simulink model "MLP_Control_Of_Induction_Motor"  (R2025b)
settings: Solver=FixedStepAuto  StartTime=0.0  StopTime=7.5  FixedStep=Ts  MaxStep=1e-3  RelTol=1e-3  EnableMultiTasking=on
PreLoadFcn:
  | IMDriveSensorData
values from neighbouring files (symbols this model uses):
  fn = 50    [Model_and_motor_parameters_for_FOC.m]
  Ibase = Pn/(1.5*Vbase)    [Model_and_motor_parameters_for_FOC.m]
  Lm = 2.717    [Model_and_motor_parameters_for_FOC.m]
  p = 2    [Model_and_motor_parameters_for_FOC.m]
  Tbase = Pn/(wbase/p)    (= 1044.05642668)    [Model_and_motor_parameters_for_FOC.m]
  Ts = 5e-6    (= 5e-06)    [Model_and_motor_parameters_for_FOC.m]
  Tsc = 1/(fsw*10)    (= 5e-05)    [Model_and_motor_parameters_for_FOC.m]
  Vbase = Vn/sqrt(3)*sqrt(2)    [Model_and_motor_parameters_for_FOC.m]
  Xls = Lls*Zbase    [Model_and_motor_parameters_for_FOC.m]
undefined symbols (not defined in the file or in its folder): ee
libraries: nesl_utility x11, ee_lib x8, fl_lib x5, eePwmGeneratorTwoLevel x1, eeTransforms x1, eeAsmFluxObserver x1, SignalEditorBlockLib x1
CloseFcn:
  | clear simlog_IMDriveSensor
  | clear logsout_IMDriveSensor
Description:
  | Three-Phase Asynchronous Drive with Sensor Control
settings Model: SimulationMode=accelerator  Creator=The MathWorks, Inc.  LastModifiedBy=Harish
settings SolverCC: AlgebraicLoopSolver=TrustRegion  AutoInsertRateTranBlk=on
settings DataIOCC: MaxDataPoints=510000  SaveOperatingPoint=on  SaveFormat=StructureWithTime  SaveOutput=off  SaveTime=off  ReturnWorkspaceOutputs=off
settings OptimizationCC: ReuseModelBlockBuffer=off  ExpressionDepthLimit=2147483647.0  LifeSpan=inf
settings DebuggingCC: AlgebraicLoopMsg=error  UnderspecifiedInitializationDetection=Classic  MergeDetectMultiDrivingBlocksExec=none  SolverPrmCheckMsg=warning  MultiTaskRateTransMsg=warning  UnconnectedInputMsg=warning  UnconnectedOutputMsg=warning  UnconnectedLineMsg=warning  StateNameClashWarn=warning  SFUnexpectedBacktrackingDiag=warning  SFNoUnconditionalDefaultTransitionDiag=warning  SFExecutionAtInitializationDiag=none  ArithmeticOperatorsInVariantConditions=warning
settings HardwareCC: ProdBitPerPointer=32.0  ProdBitPerSizeT=32.0  ProdBitPerPtrDiffT=32.0  ProdLargestAtomicFloat=None  ProdIntDivRoundTo=Undefined  ProdEndianess=Unspecified  ProdWordSize=32.0  ProdHWDeviceType=32-bit Generic
settings ModelReferenceCC: EnableRefExpFcnMdlSchedulingChecks=on  PropagateSignalLabelsOutOfModel=off
settings SFSimCC: SimUseLocalCustomCode=off  CustomCodeUndefinedFunction=UseInterfaceOnly
settings RTWCC: RTWUseLocalCustomCode=off  GPUComputeCapability=3.5  DLArmComputeVersion=19.05
settings CodeAppCC: StateflowObjectComments=on
settings GRTTargetCC: TargetLangStandard=C89/C90 (ANSI)
settings ConfigComp: CovMetricSettings=dw  CovSaveCumulativeToWorkspaceVar=on  CovSaveSingleToWorkspaceVar=on  CovExternalEMLEnable=off  CovSFcnEnable=off
settings SimscapeCC: SimscapeLogType=all  SimscapeLogSimulationStatistics=on  SimscapeLogName=simlog_IMDriveSensor  SimscapeLogDecimation=5.0  SimscapeLogLimitData=off  SimscapeLogDataHistory=510000.0

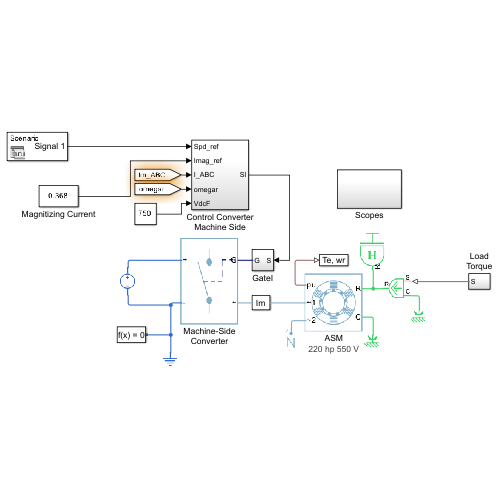
[thumbnail: Simulink's stored preview of the top-level diagram]
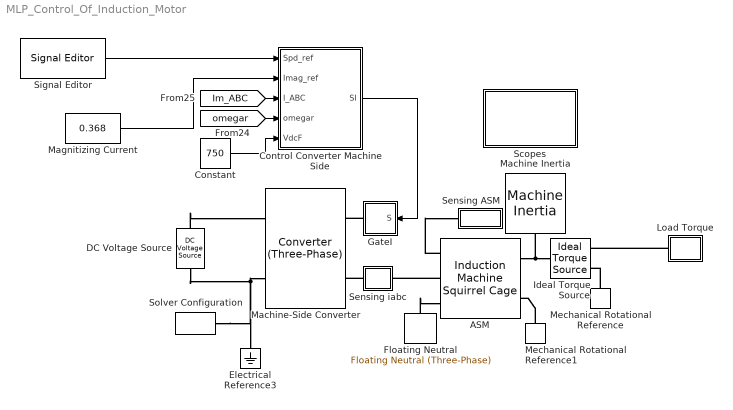
== system MLP_Control_Of_Induction_Motor ==
  ASM : ee_lib/Electromechanical/Asynchronous/Induction Machine Squirrel Cage  port_option=ee.enum.threePhasePort.composite  SRated=Pn V*A  VRated=Vn V  FRated=fn Hz  nPolePairs=p  param_unit=ee.enum.unit.si  squirrel_cage=ee.enum.squirrelcage.Single  zero_sequence=ee.enum.park.zerosequence.include  initialization_option=ee.enum.asm.initialization.fluxvariables  Rs=Rss Ohm  Xls=Xls Ohm  pu_Rs=0.0258  pu_Lls=0.0413  Rrd=Rrr Ohm  Xlrd=Xlr Ohm  pu_Rrd=0.0145  pu_Llrd=0.0424  Rrd1=0.28 Ohm  Xlrd1=0.82 Ohm  Rrd2=0.28 Ohm  Xlrd2=0.82 Ohm  pu_Rrd1=0.0290  pu_Llrd1=0.0848  pu_Rrd2=0.0290  pu_Llrd2=0.0848  Xm=Xm Ohm  pu_Lm=1.7562  X0=Xls Ohm  pu_L0=0.0413  saturation_option=0  saturation_i=[0, 4, 9, 18, 25, 34, 50, 68, 95, 120] A  saturation_v=[0, 88, 154, 198, 220, 242, 264, 286, 308, 330] V  pu_saturation_i=[0, .176, .396, .792, 1.1, 1.496, 2.2, 2.992, 4.18, 5.28]  pu_saturation_v=[0, .4, .7, .9, 1, 1.1, 1.2, 1.3, 1.4, 1.4864]  connection_option=int32(ee.enum.Connection.delta)  angular_position_specify=off  angular_position_priority=None  angular_position=0 deg  angular_position_nominal_specify=off  angular_position_nominal_value=1  angular_position_nominal_unit=deg  pu_psids_specify=off  pu_psids_priority=None  pu_psids=0  pu_psids_nominal_specify=off  pu_psids_nominal_value=1  pu_psids_nominal_unit=1  pu_psiqs_specify=off  pu_psiqs_priority=None  pu_psiqs=0  pu_psiqs_nominal_specify=off  pu_psiqs_nominal_value=1  pu_psiqs_nominal_unit=1  pu_psi0s_specify=off  pu_psi0s_priority=None  pu_psi0s=0  pu_psi0s_nominal_specify=off  pu_psi0s_nominal_value=1  pu_psi0s_nominal_unit=1  pu_psidr_specify=off  pu_psidr_priority=None  pu_psidr=0  pu_psidr_nominal_specify=off  pu_psidr_nominal_value=1  pu_psidr_nominal_unit=1  pu_psiqr_specify=off  pu_psiqr_priority=None  pu_psiqr=0  pu_psiqr_nominal_specify=off  pu_psiqr_nominal_value=1  pu_psiqr_nominal_unit=1  pu_psidr1_specify=off  pu_psidr1_priority=None  pu_psidr1=0  pu_psidr1_nominal_specify=off  pu_psidr1_nominal_value=1  pu_psidr1_nominal_unit=1  pu_psiqr1_specify=off  pu_psiqr1_priority=None  pu_psiqr1=0  pu_psiqr1_nominal_specify=off  pu_psiqr1_nominal_value=1  pu_psiqr1_nominal_unit=1  pu_psidr2_specify=off  pu_psidr2_priority=None  pu_psidr2=0  pu_psidr2_nominal_specify=off  pu_psidr2_nominal_value=1  pu_psidr2_nominal_unit=1  pu_psiqr2_specify=off  pu_psiqr2_priority=None  pu_psiqr2=0  pu_psiqr2_nominal_specify=off  pu_psiqr2_nominal_value=1  pu_psiqr2_nominal_unit=1  psids_specify=off  psids_priority=None  psids=0 Wb  psids_nominal_specify=off  psids_nominal_value=1  psids_nominal_unit=Wb  psiqs_specify=off  psiqs_priority=None  psiqs=0 Wb  psiqs_nominal_specify=off  psiqs_nominal_value=1  psiqs_nominal_unit=Wb  psi0s_specify=off  psi0s_priority=None  psi0s=0 Wb  psi0s_nominal_specify=off  psi0s_nominal_value=1  psi0s_nominal_unit=Wb  psidr_specify=off  psidr_priority=None  psidr=0 Wb  psidr_nominal_specify=off  psidr_nominal_value=1  psidr_nominal_unit=Wb  psiqr_specify=off  psiqr_priority=None  psiqr=0 Wb  psiqr_nominal_specify=off  psiqr_nominal_value=1  psiqr_nominal_unit=Wb  psidr1_specify=off  psidr1_priority=None  psidr1=0 Wb  psidr1_nominal_specify=off  psidr1_nominal_value=1  psidr1_nominal_unit=Wb  psiqr1_specify=off  psiqr1_priority=None  psiqr1=0 Wb  psiqr1_nominal_specify=off  psiqr1_nominal_value=1  psiqr1_nominal_unit=Wb  psidr2_specify=off  psidr2_priority=None  psidr2=0 Wb  psidr2_nominal_specify=off  psidr2_nominal_value=1  psidr2_nominal_unit=Wb  psiqr2_specify=off  psiqr2_priority=None  psiqr2=0 Wb  psiqr2_nominal_specify=off  psiqr2_nominal_value=1  psiqr2_nominal_unit=Wb  slip_specify=off  slip_priority=None  slip=0  slip_nominal_specify=off  slip_nominal_value=1  slip_nominal_unit=1  real_power_generated_specify=off  real_power_generated_priority=None  real_power_generated=0 W  real_power_generated_nominal_specify=off  real_power_generated_nominal_value=1  real_power_generated_nominal_unit=W  mechanical_power_consumed_specify=off  mechanical_power_consumed_priority=None  mechanical_power_consumed=0 W  mechanical_power_consumed_nominal_specify=off  mechanical_power_consumed_nominal_value=1  mechanical_power_consumed_nominal_unit=W  Tmeas=298.15 K  alpha=3.93e-3 1/K  alpha_cage=4.4e-3 1/K  stator_thermal_mass=100 J/K  rotor_thermal_mass=200 J/K  temperatureA_specify=off  temperatureA_priority=High  temperatureA=25 degC  temperatureA_nominal_specify=off  temperatureA_nominal_value=1  temperatureA_nominal_unit=degC  temperatureB_specify=off  temperatureB_priority=High  temperatureB=25 degC  temperatureB_nominal_specify=off  temperatureB_nominal_value=1  temperatureB_nominal_unit=degC  temperatureC_specify=off  temperatureC_priority=High  temperatureC=25 degC  temperatureC_nominal_specify=off  temperatureC_nominal_value=1  temperatureC_nominal_unit=degC  temperatureR_specify=off  temperatureR_priority=High  temperatureR=25 degC  temperatureR_nominal_specify=off  temperatureR_nominal_value=1  temperatureR_nominal_unit=degC
      settings: AttributesFormatString=220 hp 550 V  InternalSimscapePortConfiguration="{\"Bottom\":[],\"Left\":[{\"id\":\"R\",\"label\":\"R\",\"type\":\"foundation.mechanical.rotational.rotational\"},{\"id\":\"C\",\"label\":\"C\",\"type\":\"foundation.mechanical.rotational.rotational\"}],\"Right\":[{\"id\":\"pu_output\",\"label\":\"pu\",\"type\":\"output\"},{\"id\":\"N1\",\"label\":\"~1\",\"type\":\"foundation.electrical.three_phase\"},{\"id\":\"N2\",\"label\":\"~2\",\"type\":\"foundation.electrical.three_phase\"}],\"Top\":[]}"
  Constant : Constant  Value=750
  Control Converter Machine Side : Subsystem
  DC Voltage Source : fl_lib/Electrical/Electrical Sources/DC Voltage Source  v0=750 V
  Electrical Reference3 : fl_lib/Electrical/Electrical Elements/Electrical Reference
  Floating Neutral : ee_lib/Connectors & References/Floating Neutral (Three-Phase)  G_parasitic=1e-12 1/Ohm
      settings: InternalSimscapePortConfiguration="{\"Bottom\":[],\"Left\":[{\"id\":\"N\",\"label\":\"~\",\"type\":\"foundation.electrical.three_phase\"}],\"Right\":[],\"Top\":[]}"
  GateI : Subsystem
  Ideal Torque Source : fl_lib/Mechanical/Mechanical Sources/Ideal Torque Source
  Load Torque : Subsystem
  Machine Inertia : ee_lib/Electromechanical/Mechanical/Machine Inertia  SRated=Pn V*A  FRated=fn Hz  nPolePairs=p  inertia_option=2  J=27548 kg*m^2  H=H s*W/V/A  damper_option=2  D=39.0509 N*m/(rad/s)  pu_D=F  initialization_option=2  fMechanical0=60 Hz  fElectrical0=0 Hz
      settings: InternalSimscapePortConfiguration="{\"Bottom\":[],\"Left\":[{\"id\":\"R\",\"label\":\"R\",\"type\":\"foundation.mechanical.rotational.rotational\"}],\"Right\":[],\"Top\":[]}"
  Machine-Side Converter : ee_lib/Semiconductors & Converters/Converters/Converter (Three-Phase)  port_option=ee.enum.threePhasePort.composite  fidelity_option=ee.enum.converters.fidelity.detailed  device_type=ee.enum.converters.switchingdevice.mosfet  showThermalPort=false  K=0  Vth=0.5 V  Vgt=1 V  Vgt_off=-1 V  Ih=1 A  Vf=0.8 V  Ron=0.001 Ohm  Rds=0.001 Ohm  Goff=1e-5 1/Ohm  Eon_scalar=22.86e-3 J  Eoff_scalar=17.14e-3 J  Eoff_natural_commutation=10e-3 J  Voff=300 V  Iout_scalar=600 A  onCurrentMeasDelay=0 s  useCurrentFromPreviousCycle=false  useVoltageFromPreviousCycle=false  diode_param=2  diode_Vf=0.8 V  diode_Ron=0.001 Ohm  diode_Goff=1e-5 1/Ohm  diode_C=50 nF  diode_iRM=-235 A  diode_iF=300 A  diode_idot=-50 A/us  diode_trr_param=1  diode_trr_factor=3  diode_trr=15 us  diode_Qrr=1.5e+3 s*uA  diode_rec_loss_model=ee.enum.diode.reverseRecoveryModel.fixed  diode_ErecVal=0 J  diode_scaleWithIandV=false  diode_ErecMat=zeros(2, 3) J  diode_TjrecVec=[298.15, 398.15] K  diode_IfrecVec=[.1, 1, 10] A  diode_IrecVal=10 A  diode_VrecVal=10 V  diode_tFilter=1 / 1000 / 100 s  thermal_network_parameterization=ee.enum.thermalNetworkTopology.external  Rth=[.08, .5] K/W  Rth_Cauer=[.08, .1, .5] K/W  Rth_Foster=[.08, .14, .22, .16] K/W  thermal_mass_parameterization=ee.enum.thermalNetwork.timeconstant  thermal_mass=[.01, .5] J/K  thermal_mass_Cauer=[.01, .1, .5] J/K  thermal_mass_Foster=[.001, .005, .05, .5] J/K  thermal_time_constant=[.001, .2] s  thermal_time_constant_Cauer=[.001, .1, .2] s  thermal_time_constant_Foster=[7e-05, .0007, .01, .08] s  thermal_mass_initial_temperatures=[25, 25] degC  thermal_mass_initial_temperatures_Cauer=[25, 25, 25] degC  junction_thermal_mass=0.01 J/K  Tvec_initial_Foster=[25, 25, 25, 25] degC  snubber_type=0  Cs=1e-7 F  Rs=0.1 Ohm  Vce_loss=[0, 150, 300] V
  Magnitizing Current : Constant  Value=0.368
  Mechanical Rotational Reference : fl_lib/Mechanical/Rotational Elements/Mechanical Rotational Reference
  Mechanical Rotational Reference1 : fl_lib/Mechanical/Rotational Elements/Mechanical Rotational Reference
  Scopes : Subsystem
  Sensing ASM : Subsystem
      mask Display: disp('Te, wr')
  Sensing iabc : Subsystem
      mask Display: disp('Im')
  Signal Editor : SignalEditorBlockLib/Signal Editor  FileName=Speed_step_up.mat  ActiveScenario=Scenario  ActiveSignal=Signal 1  IsBus=off  OutputBusObjectStr=Bus: BusObject  SampleTime=0  Interpolate=off  ZeroCross=off  OutputAfterFinalValue=Setting to zero  Unit=inherit  PreserveSignalName=on  ApplySigPropsToAllScenarios=on  ApplySigPropsToAllSignals=off  SignalPropertySource=Dialog parameters
  Solver Configuration : nesl_utility/Solver Configuration  PhysicalDomain=network_engine_domain  SubClassName=solver  LeftPortType=input  RightPortType=generic  Tones=[]  Harmonics=[]  SimulateNoise=off  Profile=off  UseLocalSampling=off  EnableSwitchedLinearOptims=on  FrequencyDomain=off  UseCCode=off  RelTol=0.001  AbsTol=1e-06  MinStep=1e-09  ToWorkspace=off  RevertToSquareIcSolve=off  NumHomotopyIterations=100  PhasorMode=off  PhasorModeNumHarmonics=1  ConsistencySolver=NEWTON_FTOL  IndexReductionMethod=DerivativeReplacement  DoDC=off  ResidualTolerance=1e-09  ConsistencyTolSource=GLOBAL  ConsistencyAbsTol=0.001  ConsistencyRelTol=0.001  ConsistencyTolFactor=0.001  UseLocalSolver=on  LocalSolverChoice=NE_BACKWARD_EULER_ADVANCER  ResolveIndetEquations=on  FunctionEvalNumThread=1  LocalSolverSampleTime=Ts  DoFixedCost=on  MaxNonlinIter=5  MaxModeIter=2  ComputeImpulses=off  ImpulseIterations=2  LinearAlgebra=auto  LinearAlgebraNumThread=0  EquationFormulation=NE_TIME_EF  DelaysMemoryBudget=1024  AutomaticFiltering=on  FilteringTimeConstant=0.001  PartitionStorageMethod=AS_NEEDED  PartitionMemoryBudget=1024  PartitionMethod=FAST  MultibodyUseLocalSolver=off  MultibodyLocalSolverChoice=ODE1  MultibodyLocalSolverSampleTime=0.001
  wires:
  Control Converter Machine Side/1(SI) -> GateI/1(S)
  Magnitizing Current/1 -> Control Converter Machine Side/2(Imag_ref)
  [Im_ABC] -> Control Converter Machine Side/3(I_ABC)
  [omegar] -> Control Converter Machine Side/4(omegar)
  Constant/1 -> Control Converter Machine Side/5(VdcF)
  Signal Editor/1 -> Control Converter Machine Side/1(Spd_ref)
  connections:
  Solver Configuration/RConn1 -- Electrical Reference3/LConn1 -- DC Voltage Source/RConn1 -- Machine-Side Converter/RConn2
  Sensing iabc/LConn1 -- Machine-Side Converter/LConn2
  ASM/RConn2 -- Sensing iabc/RConn1
  ASM/LConn1 -- Machine Inertia/LConn1 -- Ideal Torque Source/LConn1
  Mechanical Rotational Reference/LConn1 -- Ideal Torque Source/RConn2
  GateI/RConn1 -- Machine-Side Converter/LConn1
  Floating Neutral/LConn1 -- ASM/RConn3
  Mechanical Rotational Reference1/LConn1 -- ASM/LConn2
  ASM/RConn1 -- Sensing ASM/RConn1
  DC Voltage Source/LConn1 -- Machine-Side Converter/RConn1
  Load Torque/RConn1 -- Ideal Torque Source/RConn1

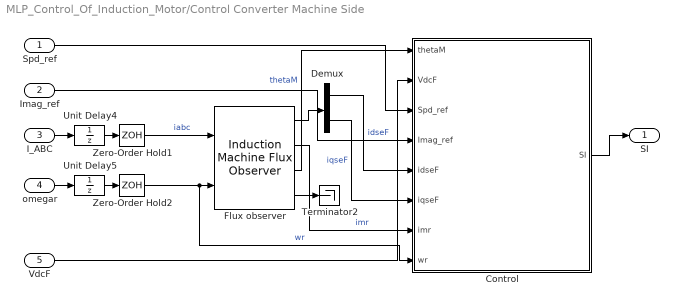
== system MLP_Control_Of_Induction_Motor/Control Converter Machine Side ==
  Spd_ref : Inport
  Imag_ref : Inport  Port=2
  I_ABC : Inport  Port=3
  omegar : Inport  Port=4
  VdcF : Inport  Port=5
  Control : Subsystem
  Demux : Demux  Outputs=2
  Flux observer : eeAsmFluxObserver/Induction Machine Flux Observer  fn=fn  Rr=Rr  Llr=Llr  Lm=Lm  Tc=1e-4  Ts=Tsc
  Terminator2 : Terminator
  Unit Delay4 : UnitDelay  SampleTime=Ts  HasFrameUpgradeWarning=on
  Unit Delay5 : UnitDelay  SampleTime=Ts  HasFrameUpgradeWarning=on
  Zero-Order Hold1 : ZeroOrderHold  SampleTime=Tsc
  Zero-Order Hold2 : ZeroOrderHold  SampleTime=Tsc
  SI : Outport  VectorParamsAs1DForOutWhenUnconnected=off
  wires:
  Zero-Order Hold1/1 -> Flux observer/1  "iabc"
  Flux observer/1 -> Demux/1
  Flux observer/4 -> Terminator2/1
  Flux observer/3 -> Control/1(thetaM)  "thetaM"
  Zero-Order Hold2/1 -> Control/8(wr), Flux observer/2  "wr"
  VdcF/1 -> Control/2(VdcF)
  Control/1(SI) -> SI/1
  Unit Delay5/1 -> Zero-Order Hold2/1
  omegar/1 -> Unit Delay5/1
  Unit Delay4/1 -> Zero-Order Hold1/1
  I_ABC/1 -> Unit Delay4/1
  Demux/1 -> Control/5(idseF)  "idseF"
  Spd_ref/1 -> Control/3(Spd_ref)
  Imag_ref/1 -> Control/4(Imag_ref)
  Demux/2 -> Control/6(iqseF)  "iqseF"
  Flux observer/2 -> Control/7(imr)  "imr"

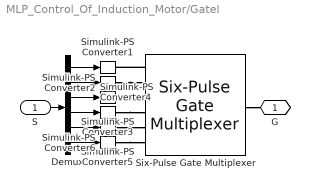
== system MLP_Control_Of_Induction_Motor/GateI ==
  S : Inport
  Demux : Demux  Outputs=6
  Simulink-PS Converter{1..6} (6 alike) : nesl_utility/Simulink-PS Converter  PhysicalDomain=network_engine_domain  SubClassName=ps_input  LeftPortType=input  RightPortType=output  PseudoPeriodic=off  Frequencies=[]  NoiseDistribution=none  NoiseParameters=[]  Unit=1  AffineConversion=off  FilteringAndDerivatives=zero  SimscapeFilterOrder=1  InputFilterTimeConstant=0.001  UdotUserProvided=1
  Six-Pulse Gate Multiplexer : ee_lib/Semiconductors & Converters/Converters/Six-Pulse Gate Multiplexer  port_option=ee.enum.controlport.ps
  G : PMIOPort  Side=Right
  wires:
  Demux/3 -> Simulink-PS Converter3/1
  Demux/6 -> Simulink-PS Converter6/1
  Demux/5 -> Simulink-PS Converter5/1
  S/1 -> Demux/1
  Demux/2 -> Simulink-PS Converter2/1
  Demux/1 -> Simulink-PS Converter1/1
  Demux/4 -> Simulink-PS Converter4/1
  connections:
  Six-Pulse Gate Multiplexer/RConn1 -- G/RConn1
  Six-Pulse Gate Multiplexer/LConn1 -- Simulink-PS Converter1/RConn1
  Simulink-PS Converter5/RConn1 -- Six-Pulse Gate Multiplexer/LConn5
  Simulink-PS Converter6/RConn1 -- Six-Pulse Gate Multiplexer/LConn6
  Simulink-PS Converter3/RConn1 -- Six-Pulse Gate Multiplexer/LConn3
  Simulink-PS Converter2/RConn1 -- Six-Pulse Gate Multiplexer/LConn2
  Simulink-PS Converter4/RConn1 -- Six-Pulse Gate Multiplexer/LConn4

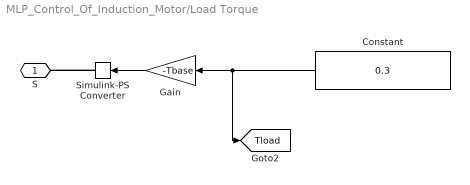
== system MLP_Control_Of_Induction_Motor/Load Torque ==
  Constant : Constant  Value=0.3
  Gain : Gain  Gain=-Tbase
  Simulink-PS Converter : nesl_utility/Simulink-PS Converter  PhysicalDomain=network_engine_domain  SubClassName=ps_input  LeftPortType=input  RightPortType=output  PseudoPeriodic=off  Frequencies=[]  NoiseDistribution=none  NoiseParameters=[]  Unit=1  AffineConversion=off  FilteringAndDerivatives=zero  SimscapeFilterOrder=1  InputFilterTimeConstant=0.001  UdotUserProvided=1
  S : PMIOPort  Side=Right
  tag scope: Tload=global
  wires:
  Gain/1 -> Simulink-PS Converter/1
  Constant/1 -> [Tload], Gain/1
  connections:
  Simulink-PS Converter/RConn1 -- S/RConn1

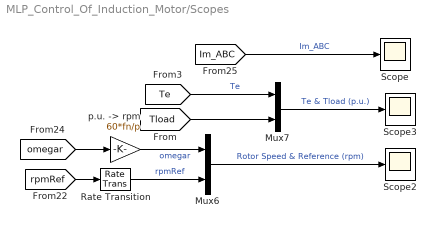
== system MLP_Control_Of_Induction_Motor/Scopes ==
  Mux6 : Mux  Inputs=2
  Mux7 : Mux  Inputs=2
  Rate Transition : RateTransition
  Scope : Scope
      settings: ActiveDisplayYMinimum=-1.7026399883890586  ActiveDisplayYMaximum=1.1439165485788876
  Scope2 : Scope
      settings: ActiveDisplayYMinimum=-192.17691683776181  ActiveDisplayYMaximum=1694.9005135340537  DataLoggingVariableName=ScopeData2
  Scope3 : Scope
      settings: ActiveDisplayYMinimum=0.11621488574308692  ActiveDisplayYMaximum=0.4685432862882189  DataLoggingVariableName=ScopeData3
  "p.u. -> rpm" : Gain  Gain=60*fn/p
  wires:
  [Im_ABC] -> Scope/1  "Im_ABC"
  Mux7/1 -> Scope3/1  "Te & Tload (p.u.)"
  Mux6/1 -> Scope2/1  "Rotor Speed & Reference (rpm)"
  [rpmRef] -> Rate Transition/1
  "p.u. -> rpm"/1 -> Mux6/1  "omegar"
  [Te] -> Mux7/1  "Te"
  [omegar] -> "p.u. -> rpm"/1
  Rate Transition/1 -> Mux6/2  "rpmRef"
  [Tload] -> Mux7/2

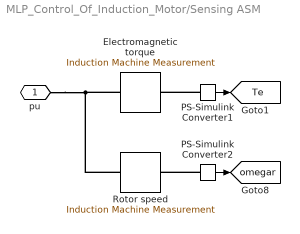
== system MLP_Control_Of_Induction_Motor/Sensing ASM ==
  Electromagnetic torque : ee_lib/Electromechanical/Asynchronous/Induction Machine Measurement  output_idx=1
      settings: InternalSimscapePortConfiguration="{\"Bottom\":[],\"Left\":[{\"id\":\"pu_input\",\"label\":\"pu\",\"type\":\"input\"}],\"Right\":[{\"id\":\"pu_output\",\"label\":\"o\",\"type\":\"output\"}],\"Top\":[]}"
  PS-Simulink Converter1 : nesl_utility/PS-Simulink Converter  PhysicalDomain=network_engine_domain  SubClassName=ps_output  LeftPortType=input  RightPortType=output  PseudoPeriodic=off  Frequencies=[]  VectorFormat=1-D array  Unit=1  AffineConversion=off
  PS-Simulink Converter2 : nesl_utility/PS-Simulink Converter  PhysicalDomain=network_engine_domain  SubClassName=ps_output  LeftPortType=input  RightPortType=output  PseudoPeriodic=off  Frequencies=[]  VectorFormat=1-D array  Unit=1  AffineConversion=off
  Rotor speed : ee_lib/Electromechanical/Asynchronous/Induction Machine Measurement  output_idx=2
      settings: InternalSimscapePortConfiguration="{\"Bottom\":[],\"Left\":[{\"id\":\"pu_input\",\"label\":\"pu\",\"type\":\"input\"}],\"Right\":[{\"id\":\"pu_output\",\"label\":\"o\",\"type\":\"output\"}],\"Top\":[]}"
  pu : PMIOPort  Side=Right
  tag scope: Te=global, omegar=global
  wires:
  PS-Simulink Converter2/1 -> [omegar]
  PS-Simulink Converter1/1 -> [Te]
  connections:
  Electromagnetic torque/LConn1 -- Rotor speed/LConn1 -- pu/RConn1
  PS-Simulink Converter1/LConn1 -- Electromagnetic torque/RConn1
  PS-Simulink Converter2/LConn1 -- Rotor speed/RConn1

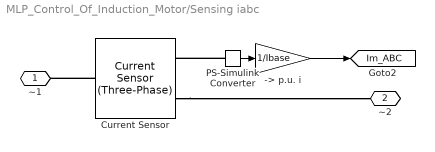
== system MLP_Control_Of_Induction_Motor/Sensing iabc ==
  -> p.u. i : Gain  Gain=1/Ibase
  Current Sensor : ee_lib/Sensors & Transducers/Current Sensor (Three-Phase)
  PS-Simulink Converter : nesl_utility/PS-Simulink Converter  PhysicalDomain=network_engine_domain  SubClassName=ps_output  LeftPortType=input  RightPortType=output  PseudoPeriodic=off  Frequencies=[]  VectorFormat=1-D array  Unit=1  AffineConversion=off
  ~1 : PMIOPort  Side=Left
  ~2 : PMIOPort  Port=2  Side=Right
  tag scope: Im_ABC=global
  wires:
  PS-Simulink Converter/1 -> -> p.u. i/1
  -> p.u. i/1 -> [Im_ABC]
  connections:
  Current Sensor/LConn1 -- ~1/RConn1
  PS-Simulink Converter/LConn1 -- Current Sensor/RConn1
  Current Sensor/RConn2 -- ~2/RConn1

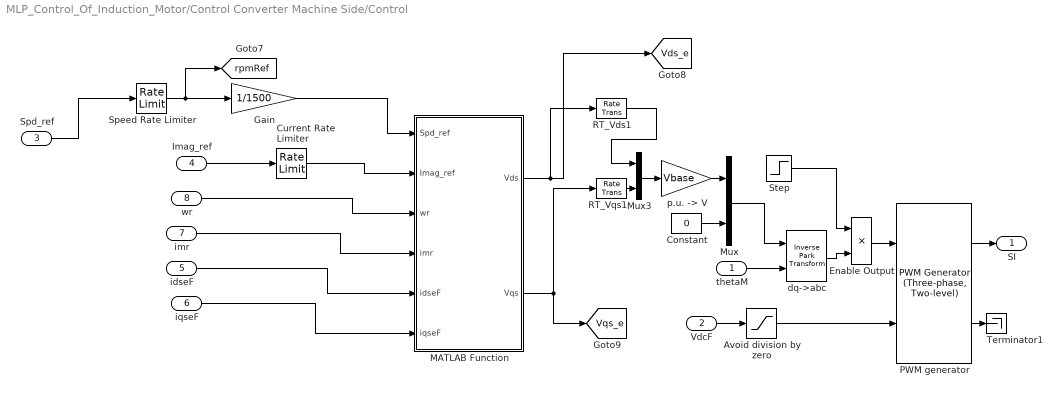
== system MLP_Control_Of_Induction_Motor/Control Converter Machine Side/Control ==
  thetaM : Inport
  VdcF : Inport  Port=2
  Spd_ref : Inport  Port=3
  Imag_ref : Inport  Port=4
  idseF : Inport  Port=5
  iqseF : Inport  Port=6
  imr : Inport  Port=7
  wr : Inport  Port=8
  Avoid division by zero : Saturate  UpperLimit=1e6  LowerLimit=10
  Constant : Constant  Value=0  SampleTime=Tsc
  Current Rate Limiter : RateLimiter  RisingSlewLimit=1/Lm*2  FallingSlewLimit=-1/Lm*2  SampleTimeMode=inherited
      settings: AttributesFormatString=2 p.u./s
  Enable Output : Product
  Gain : Gain  Gain=1/1500
  MATLAB Function : MATLAB Function  TreatAsAtomicUnit=on
  Mux : Mux  Inputs=2
  Mux3 : Mux  Inputs=2
  PWM generator : eePwmGeneratorTwoLevel/PWM Generator (Three-phase, Two-level)  PWMMode=Continuous PWM (CPWM)  CPWMMode=SVM: space vector modulation  DPWMMode=60 DPWM: 60 degree discontinuous PWM  fsw=fsw  Ts=Ts
  RT_Vds1 : RateTransition
  RT_Vqs1 : RateTransition
  Speed Rate Limiter : RateLimiter  RisingSlewLimit=2000  FallingSlewLimit=-2000  SampleTimeMode=inherited
      settings: AttributesFormatString=%<RisingSlewLimit> rpm/s
  Step : Step  Time=0  SampleTime=Ts
      settings: AttributesFormatString=%<After> at %<Time> s
  Terminator1 : Terminator
  dq->abc : eeTransforms/Inverse Park Transform  AxisAlignment=Q-axis  PowerInvariant=off
  "p.u. -> V" : Gain  Gain=Vbase
  SI : Outport  VectorParamsAs1DForOutWhenUnconnected=off
  tag scope: Vds_e=global, Vqs_e=global, rpmRef=global
  wires:
  "p.u. -> V"/1 -> Mux/1
  Step/1 -> Enable Output/1
  Avoid division by zero/1 -> PWM generator/2
  PWM generator/2 -> Terminator1/1
  Constant/1 -> Mux/2
  VdcF/1 -> Avoid division by zero/1
  thetaM/1 -> dq->abc/2
  PWM generator/1 -> SI/1
  Enable Output/1 -> PWM generator/1
  dq->abc/1 -> Enable Output/2
  Mux/1 -> dq->abc/1
  RT_Vds1/1 -> Mux3/1
  RT_Vqs1/1 -> Mux3/2
  Mux3/1 -> "p.u. -> V"/1
  MATLAB Function/1(Vds) -> [Vds_e], RT_Vds1/1
  Spd_ref/1 -> Speed Rate Limiter/1
  imr/1 -> MATLAB Function/4(imr)
  wr/1 -> MATLAB Function/3(wr)
  idseF/1 -> MATLAB Function/5(idseF)
  iqseF/1 -> MATLAB Function/6(iqseF)
  Imag_ref/1 -> Current Rate Limiter/1
  Speed Rate Limiter/1 -> Gain/1, [rpmRef]
  Gain/1 -> MATLAB Function/1(Spd_ref)
  MATLAB Function/2(Vqs) -> RT_Vqs1/1, [Vqs_e]
  Current Rate Limiter/1 -> MATLAB Function/2(Imag_ref)

== matlab function MLP_Control_Of_Induction_Motor/Control Converter Machine Side/Control/MATLAB Function ==
  data: Spd_ref input; Vds output; Imag_ref input; wr input; imr input; idseF input; iqseF input; Vqs output
function [Vds, Vqs] = foc_neural_controller(Spd_ref, Imag_ref, wr, imr, idseF, iqseF)
%#codegen

persistent w0 b0 gamma1 beta1
persistent w3 b3 gamma4 beta4
persistent w6 b6 gamma7 beta7
persistent w9 b9
persistent X_m X_s Y_m Y_s
persistent isInitialized
persistent int_Vqs % NEW: Memory for the integral action

if isempty(isInitialized)
    % Load weights (Ensure this file matches your current architecture)
    mat = coder.load('foc_mlp_weights_4.mat');
    
    X_m = double(mat.X_mean(:)); X_s = double(mat.X_std(:));
    Y_m = double(mat.Y_mean(:)); Y_s = double(mat.Y_std(:));
    
    w0     = double(mat.net_0_weight);  b0     = double(mat.net_0_bias(:));
    gamma1 = double(mat.net_1_weight(:)); beta1 = double(mat.net_1_bias(:));
    
    w3     = double(mat.net_3_weight);  b3     = double(mat.net_3_bias(:));
    gamma4 = double(mat.net_4_weight(:)); beta4 = double(mat.net_4_bias(:));
    
    w6     = double(mat.net_6_weight);  b6     = double(mat.net_6_bias(:));
    gamma7 = double(mat.net_7_weight(:)); beta7 = double(mat.net_7_bias(:));
    
    w9     = double(mat.net_9_weight);  b9     = double(mat.net_9_bias(:));
    
    isInitialized = true;
    int_Vqs = 0.0; % Initialize the integrator to zero on first run
end

% --- 1. INPUT PREPARATION ---
spd_err = double(Spd_ref - wr);
X = [spd_err; double(Imag_ref); double(wr); double(imr); double(idseF); double(iqseF)];

% --- 2. NORMALIZATION ---
X_norm = (X - X_m) ./ X_s;

% --- 3. FORWARD PASS (MLP) ---
% Layer 1
x1 = w0 * X_norm + b0;
mu1  = sum(x1) / 64.0;
var1 = sum((x1 - mu1).^2) / 64.0;
x1_ln   = (x1 - mu1) ./ sqrt(var1 + 1e-5);
x1_relu = max(0, x1_ln .* gamma1 + beta1);

% Layer 2
x2 = w3 * x1_relu + b3;
mu2  = sum(x2) / 64.0;
var2 = sum((x2 - mu2).^2) / 64.0;
x2_ln   = (x2 - mu2) ./ sqrt(var2 + 1e-5);
x2_relu = max(0, x2_ln .* gamma4 + beta4);

% Layer 3
x3 = w6 * x2_relu + b6;
mu3  = sum(x3) / 32.0;
var3 = sum((x3 - mu3).^2) / 32.0;
x3_ln   = (x3 - mu3) ./ sqrt(var3 + 1e-5);
x3_relu = max(0, x3_ln .* gamma7 + beta7);

% Output Layer (Linear)
Y_norm = w9 * x3_relu + b9;
Y = (Y_norm .* Y_s) + Y_m;

Vds = Y(1);
Vqs_ai = Y(2); % Store the AI's "guess" temporarily

% --- 4. INTEGRAL ACTION (Hybrid Neural-PI) ---
% Accumulate the speed error. This forces the steady-state error to exactly zero.
Ki_ai = 0.005; % Tuning gain for the integrator
int_Vqs = int_Vqs + (spd_err * Ki_ai);

% Anti-windup: Prevent the integrator from growing infinitely if the motor gets stuck
int_Vqs = max(-0.5, min(0.5, int_Vqs)); 

% Add the integral correction to the neural network's base output
Vqs = Vqs_ai + int_Vqs;

% --- 5. SOFTENED BRAKING GUARDRAIL ---
% Scale the braking gain to prevent violent torque transients
if spd_err < 0 
    kp_brake = 20.0; % Reduced from 100 for high-speed stability
    Vqs = Vqs + (spd_err * kp_brake); 
end

% --- 6. DYNAMIC CIRCULAR PHYSICAL LIMITS ---
% Define maximum allowable voltage magnitude (pu)
V_max_pu = 2.5; 

% Prioritize Vds to maintain the magnetic field
Vds = double(max(-1.2, min(0.3, Vds)));

% Calculate remaining voltage budget for Vqs ensuring Vds^2 + Vqs^2 <= V_max_pu^2
available_Vqs_sq = V_max_pu^2 - Vds^2;

if available_Vqs_sq > 0
    max_Vqs = sqrt(available_Vqs_sq);
else
    max_Vqs = 0; 
end

% Apply the dynamic limit to Vqs while respecting absolute operational limits
Vqs_upper_limit = min(2.5, max_Vqs);
Vqs_lower_limit = max(-1.5, -max_Vqs);
Vqs = double(max(Vqs_lower_limit, min(Vqs_upper_limit, Vqs)));

end
